simulink model "third"  (R2023a)
settings: Solver=FixedStepAuto  StartTime=0.0  StopTime=8  FixedStep=0.001  RelTol=1e-3
settings Model: Creator=evdokiiagalkina  LastModifiedBy=evdokiiagalkina

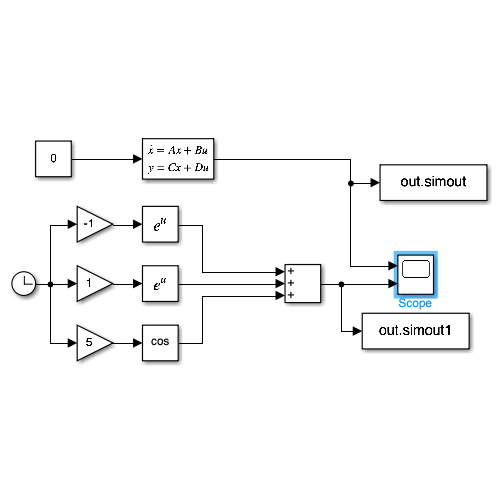
[thumbnail: Simulink's stored preview of the top-level diagram]
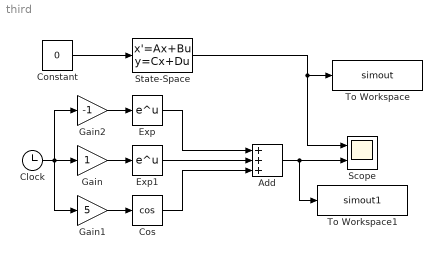
== system third ==
  Add : Sum  Inputs=+++
  Clock : Clock
  Constant : Constant  Value=0  SampleTime=-1
  Cos : Trigonometry  Operator=cos  OutputSignalType=real
  Exp : Math  OutputSignalType=real
  Exp1 : Math  OutputSignalType=real
  Gain : Gain
  Gain1 : Gain  Gain=5
  Gain2 : Gain  Gain=-1
  Scope : Scope  NumInputPorts=2
  State-Space : StateSpace  A=[1,0,0,0;0,-1,0,0;0,0,0,5;0,0,-5,0]  B=[0;0;0;0]  C=[1, 1,1, 1]  D=0  InitialCondition=[1;1;0.5;0.5]
  To Workspace : ToWorkspace  VariableName=simout  SaveFormat=Timeseries  SampleTime=-1
  To Workspace1 : ToWorkspace  VariableName=simout1  SaveFormat=Timeseries  SampleTime=-1
  wires:
  Constant/1 -> State-Space/1
  Exp/1 -> Add/1
  Exp1/1 -> Add/2
  Cos/1 -> Add/3
  Clock/1 -> Gain2/1, Gain/1, Gain1/1
  Gain2/1 -> Exp/1
  Gain1/1 -> Cos/1
  Add/1 -> Scope/2, To Workspace1/1
  Gain/1 -> Exp1/1
  State-Space/1 -> Scope/1, To Workspace/1
